simulink model "simulation_environment_R2020a"  (R2020a)
settings: Solver=ode45  StartTime=0.0  StopTime=inf  RelTol=1e-3
values from neighbouring files (symbols this model uses):
  param_initial_condition = struct()    [parameters.m]
  param_sensor = struct()    [parameters.m]
undefined symbols (not defined in the file or in its folder): param_visualization
libraries: vrlib x11, simulink_extras x1
settings Model: Creator=cha  LastModifiedBy=user
settings SolverCC: ZeroCrossAlgorithm=Adaptive
settings DataIOCC: ReturnWorkspaceOutputs=off
settings DebuggingCC: IgnoredZcDiagnostic=none  ArithmeticOperatorsInVariantConditions=warning
settings SFSimCC: SimUseLocalCustomCode=off  CustomCodeUndefinedFunction=UseInterfaceOnly
settings RTWCC: RTWUseLocalCustomCode=off

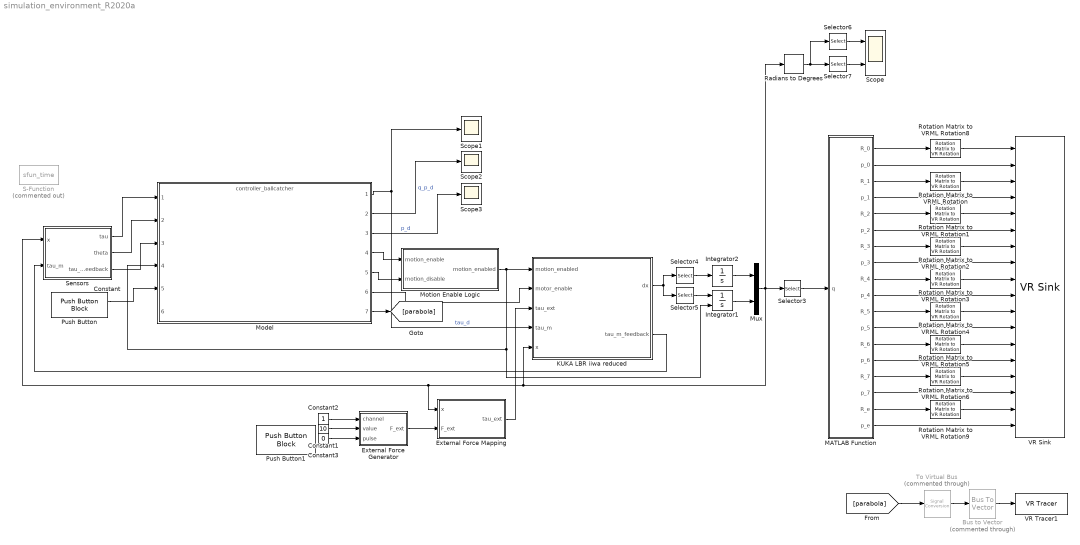
== system simulation_environment_R2020a ==
  Bus to Vector : BusToVector  Commented=through
  Constant : Constant  Value=0
  Constant1 : Constant  Value=10
  Constant2 : Constant
  Constant3 : Constant  Value=0
  External Force Generator : MATLAB Function  TreatAsAtomicUnit=on
  External Force Mapping : MATLAB Function  TreatAsAtomicUnit=on
  Integrator1 : Integrator  ExternalReset=falling  InitialCondition=[param_initial_condition.q__p_0;param_initial_condition.theta__p_0]
  Integrator2 : Integrator  InitialCondition=[param_initial_condition.q__0;param_initial_condition.theta__0]
  KUKA LBR iiwa reduced : MATLAB Function  TreatAsAtomicUnit=on
  MATLAB Function : MATLAB Function  TreatAsAtomicUnit=on
  Model : ModelReference  ModelNameDialog=controller_ballcatcher.slx  SimulationMode=Normal  ModelReferenceVersion=1.3519
  Motion Enable Logic : Subsystem
  Mux : Mux  Inputs=2
  Push Button : PushButtonBlock  ButtonText=MFT Button
  Push Button1 : PushButtonBlock  ButtonText=Force/Torque
  Radians to Degrees : simulink_extras/Transformations/Radians to Degrees
  Rotation Matrix to VRML Rotation{,1..6,8..9} (9 alike) : vrlib/Utilities/Rotation Matrix to VR Rotation  maxzero=1e-12
      settings: SourceProductBaseCode=SL
  S-Function : S-Function  Commented=on  FunctionName=sfun_time  Parameters=param_visualization.retardation  SFunctionDeploymentMode=off  EnableBusSupport=off
  Scope : Scope  NumInputPorts=2
  Scope1 : Scope
  Scope2 : Scope
  Scope3 : Scope
  Selector3 : Selector  InputPortWidth=28  IndexOptions=Index vector (dialog)  Indices=[1:7]  OutputSizes=1
  Selector4 : Selector  InputPortWidth=28  IndexOptions=Index vector (dialog)  Indices=[1:14]  OutputSizes=1
  Selector5 : Selector  InputPortWidth=28  IndexOptions=Index vector (dialog)  Indices=[15:28]  OutputSizes=1
  Selector6 : Selector  InputPortWidth=28  IndexOptions=Index vector (dialog)  Indices=[1:7]  OutputSizes=1
  Selector7 : Selector  InputPortWidth=28  IndexOptions=Index vector (dialog)  Indices=[15:21]  OutputSizes=1
  Sensors : Subsystem  TreatAsAtomicUnit=on  SystemSampleTime=param_sensor.T_a
  To Virtual Bus : SignalConversion  Commented=through  ConversionOutput=Virtual bus  OverrideOpt=off
  VR Sink : vrlib/VR Sink  InstantiateOnLoad=on  SampleTime=0.03/param_visualization.retardation  ViewEnable=on  RemoteChange=off  RemoteView=off  FieldsWritten=Robot.rotation.4.1.1.double#Robot.translation.3.1.1.double#A1.rotation.4.1.1.double#A1.translation.3.1.1.double#A2.rotation.4.1.1.double#A2.translation.3.1.1.double#A3.rotation.4.1.1.double#A3.translation.3.1.1.double#A4.rotation.4.1.1.double#A4.translation.3.1.1.double#A5.rotation.4.1.1.double#A5.translation.3.1.1.double#A6.rotation.4.1.1.double#A6.translation.3.1.1.double#A7.rotation.4.1.1.double#A7.translation.3.1.1.double#endeffector.rotation.4.1.1.double#endeffector.translation.3.1.1.double  WorldFileName=iiwa.wrl  AutoView=off  VideoDimensions=[]  AllowVariableSize=off
  VR Tracer1 : vrlib/VR Tracer  VrmlFile=iiwa.wrl  MarkerName=Box  UseLines=on  UseTriads=off  MarkerScale=[1 1 1]*1e-2  MarkerColorSelection=Selected from color list  MarkerColor=green  rgbval=[1 0 0]  Ts=0.01  ForceViewerOpen=off  ConnectPlane=off  PlaneCoeff=[0 1 0 0]  ConnectPoint=None  PointCoord=[0 0 0]
      settings: SourceProductBaseCode=SL
  wires:
  MATLAB Function/11(R_5) -> Rotation Matrix to VRML Rotation4/1
  MATLAB Function/9(R_4) -> Rotation Matrix to VRML Rotation3/1
  MATLAB Function/5(R_2) -> Rotation Matrix to VRML Rotation1/1
  MATLAB Function/15(R_7) -> Rotation Matrix to VRML Rotation6/1
  MATLAB Function/13(R_6) -> Rotation Matrix to VRML Rotation5/1
  MATLAB Function/3(R_1) -> Rotation Matrix to VRML Rotation/1
  MATLAB Function/7(R_3) -> Rotation Matrix to VRML Rotation2/1
  Sensors/1(tau) -> Model/1
  Model/1 -> Scope1/1, KUKA LBR iiwa reduced/4(tau_m)  "tau_d"
  Mux/1 -> Radians to Degrees/1, KUKA LBR iiwa reduced/5(x), External Force Mapping/1(x), Sensors/1(x), Selector3/1
  Sensors/2(theta) -> Model/2
  KUKA LBR iiwa reduced/1(dx) -> Selector4/1, Selector5/1
  Sensors/3(tau_m_feedback) -> Model/3
  External Force Mapping/1(tau_ext) -> KUKA LBR iiwa reduced/3(tau_ext)
  Integrator2/1 -> Mux/1
  Integrator1/1 -> Mux/2
  Selector4/1 -> Integrator2/1
  Selector5/1 -> Integrator1/1
  Motion Enable Logic/1(motion_enabled) -> Integrator1/2, Model/4, KUKA LBR iiwa reduced/1(motion_enabled)
  KUKA LBR iiwa reduced/2(tau_m_feedback) -> Sensors/2(tau_m)
  Selector7/1 -> Scope/2
  Selector6/1 -> Scope/1
  External Force Generator/1(F_ext) -> External Force Mapping/2(F_ext)
  Constant1/1 -> External Force Generator/2(value)
  Constant2/1 -> External Force Generator/1(channel)
  Constant3/1 -> External Force Generator/3(pulse)
  MATLAB Function/1(R_0) -> Rotation Matrix to VRML Rotation8/1
  Selector3/1 -> MATLAB Function/1(q)
  MATLAB Function/17(R_e) -> Rotation Matrix to VRML Rotation9/1
  Radians to Degrees/1 -> Selector7/1, Selector6/1
  Constant/1 -> Model/5
  Rotation Matrix to VRML Rotation9/1 -> VR Sink/17
  MATLAB Function/18(p_e) -> VR Sink/18
  Rotation Matrix to VRML Rotation8/1 -> VR Sink/1
  MATLAB Function/2(p_0) -> VR Sink/2
  Rotation Matrix to VRML Rotation/1 -> VR Sink/3
  MATLAB Function/4(p_1) -> VR Sink/4
  Rotation Matrix to VRML Rotation1/1 -> VR Sink/5
  MATLAB Function/6(p_2) -> VR Sink/6
  Rotation Matrix to VRML Rotation2/1 -> VR Sink/7
  MATLAB Function/8(p_3) -> VR Sink/8
  Rotation Matrix to VRML Rotation3/1 -> VR Sink/9
  MATLAB Function/10(p_4) -> VR Sink/10
  Rotation Matrix to VRML Rotation4/1 -> VR Sink/11
  MATLAB Function/12(p_5) -> VR Sink/12
  Rotation Matrix to VRML Rotation5/1 -> VR Sink/13
  MATLAB Function/14(p_6) -> VR Sink/14
  Rotation Matrix to VRML Rotation6/1 -> VR Sink/15
  MATLAB Function/16(p_7) -> VR Sink/16
  Model/2 -> Scope2/1  "q_p_d"
  Model/6 -> KUKA LBR iiwa reduced/2(motor_enable)
  Model/5 -> Motion Enable Logic/2(motion_disable)
  Model/4 -> Motion Enable Logic/1(motion_enable)
  Model/3 -> Scope3/1  "p_d"
  Bus to Vector/1 -> VR Tracer1/1
  [parabola] -> To Virtual Bus/1
  To Virtual Bus/1 -> Bus to Vector/1
  Model/7 -> [parabola]

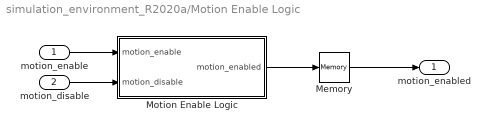
== system simulation_environment_R2020a/Motion Enable Logic ==
  motion_enable : Inport
  motion_disable : Inport  Port=2
  Memory : Memory
  Motion Enable Logic : MATLAB Function  TreatAsAtomicUnit=on
  motion_enabled : Outport  VectorParamsAs1DForOutWhenUnconnected=off
  wires:
  motion_disable/1 -> Motion Enable Logic/2(motion_disable)
  motion_enable/1 -> Motion Enable Logic/1(motion_enable)
  Motion Enable Logic/1(motion_enabled) -> Memory/1
  Memory/1 -> motion_enabled/1

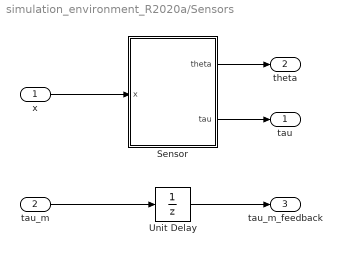
== system simulation_environment_R2020a/Sensors ==
  x : Inport
  tau_m : Inport  Port=2
  Sensor : MATLAB Function  SystemSampleTime=param_sensor.T_a
  Unit Delay : UnitDelay  SampleTime=-1  HasFrameUpgradeWarning=on
  tau : Outport  VectorParamsAs1DForOutWhenUnconnected=off
  theta : Outport  Port=2  VectorParamsAs1DForOutWhenUnconnected=off
  tau_m_feedback : Outport  Port=3  VectorParamsAs1DForOutWhenUnconnected=off
  wires:
  Sensor/1(theta) -> theta/1
  Sensor/2(tau) -> tau/1
  x/1 -> Sensor/1(x)
  tau_m/1 -> Unit Delay/1
  Unit Delay/1 -> tau_m_feedback/1

== matlab function simulation_environment_R2020a/KUKA LBR iiwa reduced ==
  data: motion_enabled input; motor_enable input; tau_ext input; tau_m input; x input; dx output; param_robot parameter; tau_m_feedback output
function [dx,tau_m_feedback]   = fcn(motion_enabled,motor_enable, tau_ext, tau_m, x, param_robot)
  if(motion_enabled)
    q=x(1:7);
    theta=x(8:14);
    q_p=x(15:21);
    theta_p=x(22:28);
    
    motor_disable=(motor_enable~=1);
    tau_m(motor_disable)=0;
    
    M=iiwa_reduced_inertia_matrix(q,param_robot);
    C=iiwa_reduced_coriolis_matrix(q,q_p,param_robot);
    N=iiwa_conservative_force(q,q_p,theta,theta_p,param_robot);
    dx=[q_p;...
      theta_p;...
      M\(tau_ext-C*q_p-N(1:7));...
      param_robot.B\(tau_m-N(8:14))];
    
    dx(repmat(motor_disable,4,1))=0;
    tau_m_feedback=tau_m;
  else
    dx=zeros(size(x));
    tau_m_feedback=zeros(size(tau_m));
  end
end

== matlab function simulation_environment_R2020a/MATLAB Function ==
  data: R_0 output; p_0 output; q input; R_1 output; p_1 output; R_2 output; p_2 output; R_3 output; p_3 output; R_4 output; p_4 output; R_5 output; p_5 output; R_6 output; p_6 output; R_7 output; p_7 output; R_e output; p_e output; param_robot parameter
function [R_0,p_0,R_1,p_1,R_2,p_2,R_3,p_3,R_4,p_4,R_5,p_5,R_6,p_6,R_7,p_7,R_e,p_e] = fcn(q,param_robot)
  p_0=param_robot.p_0;
  R_0=param_robot.R_0; 
  H=iiwa_homogeneous_transformation(q,param_robot);
  R_1=H(1:3,1:3);
  p_1=H(1:3,4);
  R_2=H(1:3,5:7);
  p_2=H(1:3,8);
  R_3=H(1:3,9:11);
  p_3=H(1:3,12);
  R_4=H(1:3,13:15);
  p_4=H(1:3,16);
  R_5=H(1:3,17:19);
  p_5=H(1:3,20);
  R_6=H(1:3,21:23);
  p_6=H(1:3,24);
  R_7=H(1:3,25:27);
  p_7=H(1:3,28);
  R_e=H(1:3,29:31);
  p_e=H(1:3,32);
end

== matlab function simulation_environment_R2020a/Sensors/Sensor ==
  settings: sampleTime=param.T_a
  data: x input; theta output; param_robot parameter; tau output
function [theta,tau] = fcn(x,param_robot)
  q=x(1:7);
  theta=x(8:14);
  tau=param_robot.K*(theta-q);
end

== matlab function simulation_environment_R2020a/Motion Enable Logic/Motion Enable Logic ==
  data: motion_enable input; motion_enabled output; motion_disable input
function motion_enabled = fcn(motion_enable, motion_disable)
  persistent x_motion_enabled;

  if(isempty(x_motion_enabled))
      x_motion_enabled=0;
  end
  
  if(motion_disable)
    x_motion_enabled=0;
  elseif(motion_enable)
    x_motion_enabled=1;
  end
  
  motion_enabled=x_motion_enabled;
end

== matlab function simulation_environment_R2020a/External Force Generator ==
  data: channel input; F_ext output; value input; pulse input
function F_ext = fcn(channel,value,pulse)
  F_ext=zeros(6,1);
  if(pulse && channel>=1 && channel<=6)
    F_ext(channel)=value;
  end
end

== matlab function simulation_environment_R2020a/External Force Mapping ==
  data: x input; F_ext input; tau_ext output; param_robot parameter
function tau_ext = fcn(x, F_ext,param_robot)
  n=7;
  q=x(1:n);
  J=iiwa_jacobian(q,param_robot);
  H=iiwa_homogeneous_transformation_endeffector(q,param_robot);
  R_0_e=H(1:3,1:3);
  tau_ext=J'*[R_0_e,zeros(3);zeros(3),R_0_e]*F_ext;
end
